simulink model "Cowley436Lab4"  (R2022b)
settings: Solver=VariableStepAuto  StartTime=0.0  StopTime=10.0  RelTol=1e-3
values from neighbouring files (symbols this model uses):
  b = 0.25    [Cowley_436HW2.m]    (also in Cowley_MME436Lab3.m = 0.1; poleIdentification.m = 2*wn*zeta; tfCharacterisitcs.m = 2)
  L = 0.5    [Cowley_MME436Lab3.m]
  R = 1    [Cowley_MME436Lab3.m]
undefined symbols (not defined in the file or in its folder): Jeq, Kb, Kt
settings Model: Creator=mattcowley  LastModifiedBy=mattcowley

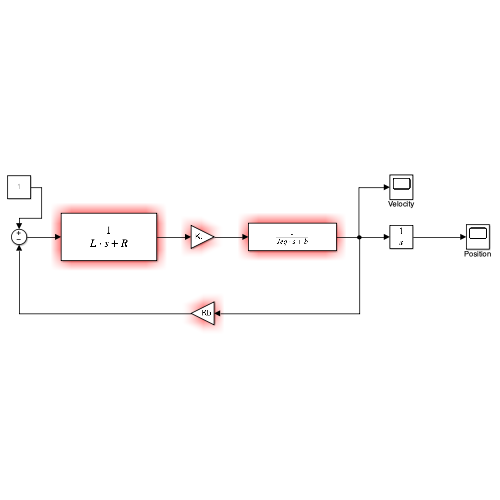
[thumbnail: Simulink's stored preview of the top-level diagram]
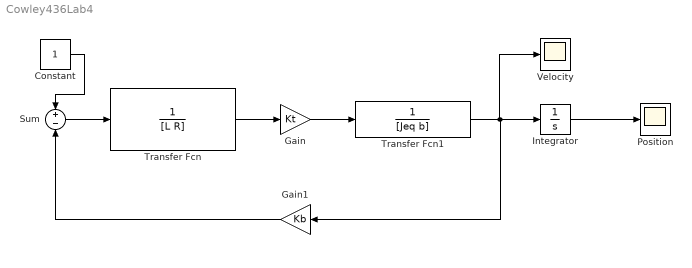
== system Cowley436Lab4 ==
  Constant : Constant
  Gain : Gain  Gain=Kt
  Gain1 : Gain  Gain=Kb
  Integrator : Integrator
  Position : Scope
  Sum : Sum  Inputs=+-
  Transfer Fcn : TransferFcn  Denominator=[L R]
  Transfer Fcn1 : TransferFcn  Denominator=[Jeq b]
  Velocity : Scope
  wires:
  Gain1/1 -> Sum/2
  Sum/1 -> Transfer Fcn/1
  Transfer Fcn/1 -> Gain/1
  Gain/1 -> Transfer Fcn1/1
  Transfer Fcn1/1 -> Velocity/1, Gain1/1, Integrator/1
  Integrator/1 -> Position/1
  Constant/1 -> Sum/1
